simulink library "psa"  (R2021b)
settings: Solver=VariableStepAuto  StartTime=0.0  StopTime=10.0  RelTol=1e-3
undefined symbols (not defined in the file or in its folder): ENUM_B2VDCCHGCONNSTA_CONNECT, ENUM_BRAKEPEDAL_PRESSED, ENUM_HVPWROFFREQ_POWEROFF, ENUM_KEYSTATUS_OFF, ENUM_KEYSTATUS_ON, ENUM_KEYSTATUS_START, ENUM_MCUFAILGRADE_SEVERE, ENUM_PEUHVILSTA_EACERROR, ENUM_PEUHVILSTA_EHPSERROR, ENUM_PEUHVILSTA_PEUERROR, ENUM_PEUSELFCHKSTS_FAULT, ENUM_PMMMODE_INITIALIZE, ENUM_TARGETGEAR_NEUTRAL, FALSE, KPMM_ChrgwakeDebon_cnt, KPSA_ActTimeEmergencySD_s, KPSA_AfterrunWaitTime_s, KPSA_AlcLockPass_ovrdflg_flg, KPSA_AlcLockPass_ovrdval_flg, KPSA_AlcLockPassTime_s, KPSA_APSPosnSafe_pct, KPSA_FakeWakeRESET_flg, KPSA_Keystatus_enum_dovrdflg, KPSA_Keystatus_enum_dovrdval, KPSA_KeystatusWaitTime_s, KPSA_PBOnTimeForEMStop_s, KPSA_PBTrigHoldtime_s, KPSA_RcvTimeEmergencySD_s, KPSA_VehspdSafe_kph, TRUE
libraries: hcu_lib x7, simulink x3
settings Model: Creator=Shawn  LastModifiedBy=FVT22063
settings SolverCC: AlgebraicLoopSolver=TrustRegion
settings DebuggingCC: SFMachineParentedDataDiag=warning

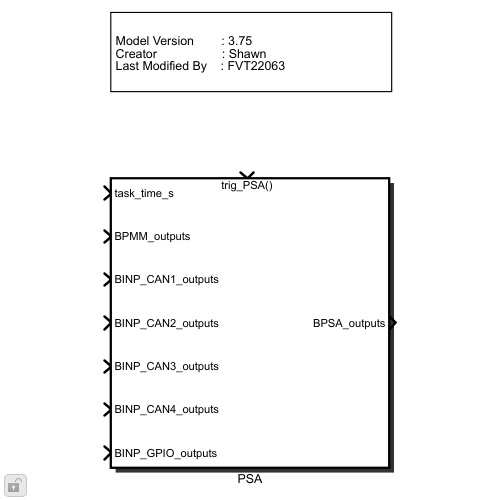
[thumbnail: Simulink's stored preview of the top-level diagram]
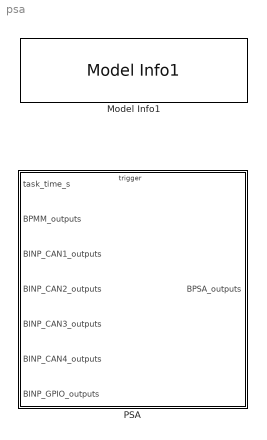
== system psa ==
  Model Info1 : hcu_lib/Model Info1  BlockCM=None  Frame=on  DisplayStringWithTags=|  HorizontalTextAlignment=Left  LeftAlignmentValue=0.02  SourceBlockDiagram=hcu_lib  TagMaxNumber=20
      | Model Version        : %<ModelVersion>
      | Creator                   : %<Creator>
      | Last Modified By    : %<LastModifiedBy>
      settings: SourceProductName=HCU Relative Block Library
  PSA : Subsystem
      settings: RTWSystemCode=Nonreusable function  RTWFcnNameOpts=Use subsystem name  RTWFileNameOpts=Use subsystem name

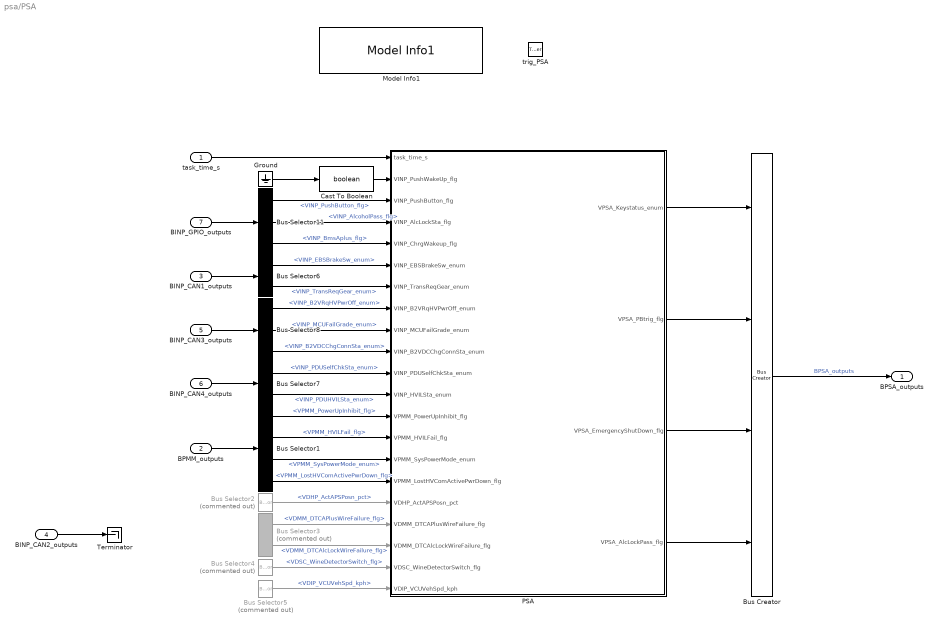
== system psa/PSA ==
  task_time_s : Inport
  BPMM_outputs : Inport  Port=2  OutDataTypeStr=Bus: BPMM_outputs
  BINP_CAN1_outputs : Inport  Port=3  OutDataTypeStr=Bus: BINP_CAN1_outputs
  BINP_CAN2_outputs : Inport  Port=4  OutDataTypeStr=Bus: BHAL_CAN2_outputs
  BINP_CAN3_outputs : Inport  Port=5  OutDataTypeStr=Bus: BINP_CAN3_outputs
  BINP_CAN4_outputs : Inport  Port=6  OutDataTypeStr=Bus: BINP_CAN4_outputs
  BINP_GPIO_outputs : Inport  Port=7  OutDataTypeStr=Bus: BINP_GPIO_outputs
  trig_PSA : TriggerPort  TriggerType=function-call  VariantControl=(inherit)
  Bus Creator : BusCreator  Inputs=4  OutDataTypeStr=Bus: BPSA_outputs  NonVirtualBus=on
  Bus Selector1 : BusSelector  OutputSignals=VPMM_PowerUpInhibit_flg,VPMM_HVILFail_flg,VPMM_SysPowerMode_enum,VPMM_LostHVComActivePwrDown_flg
  Bus Selector11 : BusSelector  OutputSignals=VINP_PushButton_flg,VINP_AlcoholPass_flg,VINP_BmsAplus_flg
  Bus Selector2 : BusSelector  Commented=on  OutputSignals=VDHP_ActAPSPosn_pct
  Bus Selector3 : BusSelector  Commented=on  OutputSignals=VDMM_DTCAPlusWireFailure_flg,VDMM_DTCAlcLockWireFailure_flg
  Bus Selector4 : BusSelector  Commented=on  OutputSignals=VDSC_WineDetectorSwitch_flg
  Bus Selector5 : BusSelector  Commented=on  OutputSignals=VDIP_VCUVehSpd_kph
  Bus Selector6 : BusSelector  OutputSignals=VINP_EBSBrakeSw_enum,VINP_TransReqGear_enum
  Bus Selector7 : BusSelector  OutputSignals=VINP_PDUSelfChkSta_enum,VINP_PDUHVILSta_enum
  Bus Selector8 : BusSelector  OutputSignals=VINP_B2VRqHVPwrOff_enum,VINP_MCUFailGrade_enum,VINP_B2VDCChgConnSta_enum
  Cast To Boolean : DataTypeConversion  OutDataTypeStr=boolean
  Ground : Ground
  Model Info1 : hcu_lib/Model Info1  BlockCM=None  Frame=on  DisplayStringWithTags=|  HorizontalTextAlignment=Left  LeftAlignmentValue=0.02  SourceBlockDiagram=hcu_lib  TagMaxNumber=20
      | Model Version        : %<ModelVersion>
      | Creator                   : %<Creator>
      | Last Modified By    : %<LastModifiedBy>
      settings: SourceProductName=HCU Relative Block Library
  PSA : Subsystem
  Terminator : Terminator
  BPSA_outputs : Outport  OutDataTypeStr=Bus: BPSA_outputs  VectorParamsAs1DForOutWhenUnconnected=off
  wires:
  Bus Selector1/1 -> PSA/13(VPMM_PowerUpInhibit_flg)  "<VPMM_PowerUpInhibit_flg>"
  Bus Creator/1 -> BPSA_outputs/1  "BPSA_outputs"
  PSA/1(VPSA_Keystatus_enum) -> Bus Creator/1
  task_time_s/1 -> PSA/1(task_time_s)
  PSA/2(VPSA_PBtrig_flg) -> Bus Creator/2
  PSA/3(VPSA_EmergencyShutDown_flg) -> Bus Creator/3
  Bus Selector2/1 -> PSA/17(VDHP_ActAPSPosn_pct)  "<VDHP_ActAPSPosn_pct>"
  Bus Selector1/2 -> PSA/14(VPMM_HVILFail_flg)  "<VPMM_HVILFail_flg>"
  PSA/4(VPSA_AlcLockPass_flg) -> Bus Creator/4
  Bus Selector1/3 -> PSA/15(VPMM_SysPowerMode_enum)  "<VPMM_SysPowerMode_enum>"
  Bus Selector1/4 -> PSA/16(VPMM_LostHVComActivePwrDown_flg)  "<VPMM_LostHVComActivePwrDown_flg>"
  Bus Selector3/1 -> PSA/18(VDMM_DTCAPlusWireFailure_flg)  "<VDMM_DTCAPlusWireFailure_flg>"
  Bus Selector3/2 -> PSA/19(VDMM_DTCAlcLockWireFailure_flg)  "<VDMM_DTCAlcLockWireFailure_flg>"
  Bus Selector4/1 -> PSA/20(VDSC_WineDetectorSwitch_flg)  "<VDSC_WineDetectorSwitch_flg>"
  Bus Selector5/1 -> PSA/21(VDIP_VCUVehSpd_kph)  "<VDIP_VCUVehSpd_kph>"
  BPMM_outputs/1 -> Bus Selector1/1
  BINP_CAN1_outputs/1 -> Bus Selector6/1
  Bus Selector6/1 -> PSA/6(VINP_EBSBrakeSw_enum)  "<VINP_EBSBrakeSw_enum>"
  BINP_CAN4_outputs/1 -> Bus Selector7/1
  Bus Selector7/2 -> PSA/12(VINP_HVILSta_enum)  "<VINP_PDUHVILSta_enum>"
  BINP_CAN3_outputs/1 -> Bus Selector8/1
  Bus Selector7/1 -> PSA/11(VINP_PDUSelfChkSta_enum)  "<VINP_PDUSelfChkSta_enum>"
  Bus Selector8/1 -> PSA/8(VINP_B2VRqHVPwrOff_enum)  "<VINP_B2VRqHVPwrOff_enum>"
  Bus Selector8/2 -> PSA/9(VINP_MCUFailGrade_enum)  "<VINP_MCUFailGrade_enum>"
  Bus Selector8/3 -> PSA/10(VINP_B2VDCChgConnSta_enum)  "<VINP_B2VDCChgConnSta_enum>"
  Bus Selector6/2 -> PSA/7(VINP_TransReqGear_enum)  "<VINP_TransReqGear_enum>"
  Ground/1 -> Cast To Boolean/1
  Cast To Boolean/1 -> PSA/2(VINP_PushWakeUp_flg)
  BINP_GPIO_outputs/1 -> Bus Selector11/1
  Bus Selector11/1 -> PSA/3(VINP_PushButton_flg)  "<VINP_PushButton_flg>"
  Bus Selector11/2 -> PSA/4(VINP_AlcLockSta_flg)  "<VINP_AlcoholPass_flg>"
  BINP_CAN2_outputs/1 -> Terminator/1
  Bus Selector11/3 -> PSA/5(VINP_ChrgWakeup_flg)  "<VINP_BmsAplus_flg>"

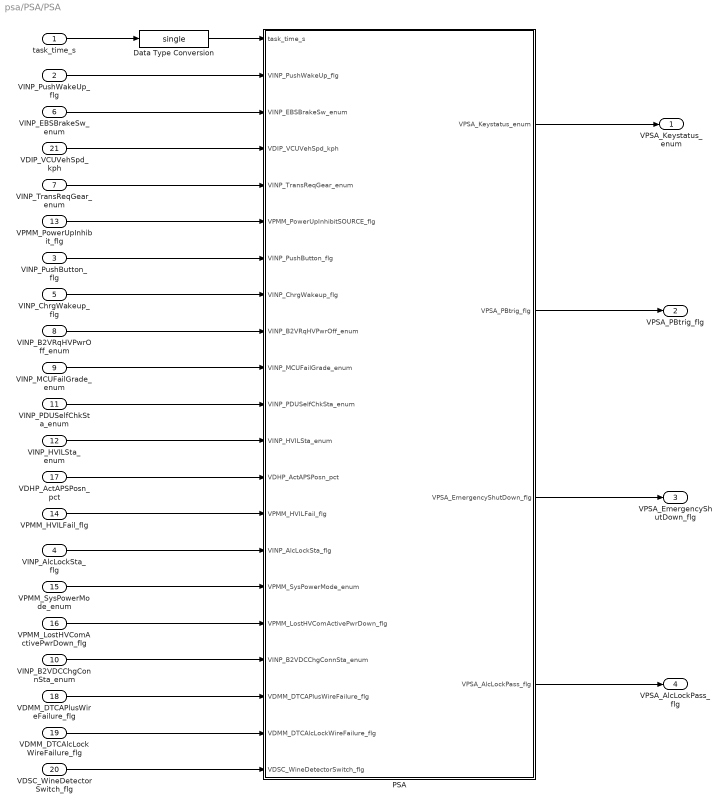
== system psa/PSA/PSA ==
  task_time_s : Inport
  VINP_PushWakeUp_flg : Inport  Port=2
  VINP_PushButton_flg : Inport  Port=3
  VINP_AlcLockSta_flg : Inport  Port=4
  VINP_ChrgWakeup_flg : Inport  Port=5
  VINP_EBSBrakeSw_enum : Inport  Port=6
  VINP_TransReqGear_enum : Inport  Port=7
  VINP_B2VRqHVPwrOff_enum : Inport  Port=8
  VINP_MCUFailGrade_enum : Inport  Port=9
  VINP_B2VDCChgConnSta_enum : Inport  Port=10
  VINP_PDUSelfChkSta_enum : Inport  Port=11
  VINP_HVILSta_enum : Inport  Port=12
  VPMM_PowerUpInhibit_flg : Inport  Port=13
  VPMM_HVILFail_flg : Inport  Port=14
  VPMM_SysPowerMode_enum : Inport  Port=15
  VPMM_LostHVComActivePwrDown_flg : Inport  Port=16
  VDHP_ActAPSPosn_pct : Inport  Port=17
  VDMM_DTCAPlusWireFailure_flg : Inport  Port=18
  VDMM_DTCAlcLockWireFailure_flg : Inport  Port=19
  VDSC_WineDetectorSwitch_flg : Inport  Port=20
  VDIP_VCUVehSpd_kph : Inport  Port=21
  Data Type Conversion : DataTypeConversion  OutDataTypeStr=single
  PSA : Subsystem  Priority=1
      settings: AttributesFormatString=< Priority = %<Priority>>
  VPSA_Keystatus_enum : Outport  VectorParamsAs1DForOutWhenUnconnected=off
  VPSA_PBtrig_flg : Outport  Port=2  VectorParamsAs1DForOutWhenUnconnected=off
  VPSA_EmergencyShutDown_flg : Outport  Port=3  VectorParamsAs1DForOutWhenUnconnected=off
  VPSA_AlcLockPass_flg : Outport  Port=4  VectorParamsAs1DForOutWhenUnconnected=off
  wires:
  VPMM_PowerUpInhibit_flg/1 -> PSA/6(VPMM_PowerUpInhibitSOURCE_flg)
  PSA/1(VPSA_Keystatus_enum) -> VPSA_Keystatus_enum/1
  VINP_PushWakeUp_flg/1 -> PSA/2(VINP_PushWakeUp_flg)
  VINP_TransReqGear_enum/1 -> PSA/5(VINP_TransReqGear_enum)
  VDIP_VCUVehSpd_kph/1 -> PSA/4("VDIP_VCUVehSpd_kph ")
  Data Type Conversion/1 -> PSA/1(task_time_s)
  VINP_PushButton_flg/1 -> PSA/7(VINP_PushButton_flg)
  VINP_EBSBrakeSw_enum/1 -> PSA/3(VINP_EBSBrakeSw_enum)
  task_time_s/1 -> Data Type Conversion/1
  VINP_ChrgWakeup_flg/1 -> PSA/8(VINP_ChrgWakeup_flg)
  PSA/2(VPSA_PBtrig_flg) -> VPSA_PBtrig_flg/1
  PSA/3(VPSA_EmergencyShutDown_flg) -> VPSA_EmergencyShutDown_flg/1
  VINP_B2VRqHVPwrOff_enum/1 -> PSA/9(VINP_B2VRqHVPwrOff_enum)
  VINP_PDUSelfChkSta_enum/1 -> PSA/11(VINP_PDUSelfChkSta_enum)
  VINP_HVILSta_enum/1 -> PSA/12(VINP_HVILSta_enum)
  VDHP_ActAPSPosn_pct/1 -> PSA/13(VDHP_ActAPSPosn_pct)
  VPMM_HVILFail_flg/1 -> PSA/14(VPMM_HVILFail_flg)
  VINP_MCUFailGrade_enum/1 -> PSA/10(VINP_MCUFailGrade_enum)
  VINP_AlcLockSta_flg/1 -> PSA/15(VINP_AlcLockSta_flg)
  PSA/4(VPSA_AlcLockPass_flg) -> VPSA_AlcLockPass_flg/1
  VPMM_SysPowerMode_enum/1 -> PSA/16(VPMM_SysPowerMode_enum)
  VPMM_LostHVComActivePwrDown_flg/1 -> PSA/17(VPMM_LostHVComActivePwrDown_flg)
  VINP_B2VDCChgConnSta_enum/1 -> PSA/18(VINP_B2VDCChgConnSta_enum)
  VDMM_DTCAPlusWireFailure_flg/1 -> PSA/19(VDMM_DTCAPlusWireFailure_flg)
  VDMM_DTCAlcLockWireFailure_flg/1 -> PSA/20(VDMM_DTCAlcLockWireFailure_flg)
  VDSC_WineDetectorSwitch_flg/1 -> PSA/21(VDSC_WineDetectorSwitch_flg)

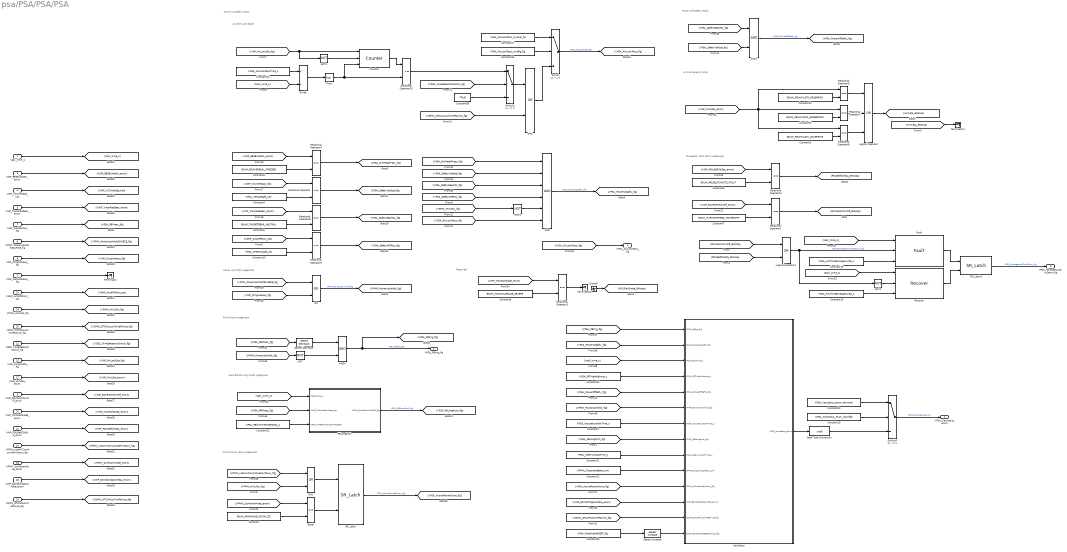
== system psa/PSA/PSA/PSA ==
  note: Push Button Judgement
  note: Active Power Down Judgement
  note: Emergency Shut Down Judgement
  note: Power Off Safety Check
  note: Reserved
  note: Push Botton Long Press Judgement
  note: Power Up Inhibit Judgement
  note: HVIL Emergency Stop
  note: Alcohol Lock State
  note: Power Up Safety Check
  task_time_s : Inport
  VINP_PushWakeUp_flg : Inport  Port=2
  VINP_EBSBrakeSw_enum : Inport  Port=3
  "VDIP_VCUVehSpd_kph " : Inport  Port=4
  VINP_TransReqGear_enum : Inport  Port=5
  VPMM_PowerUpInhibitSOURCE_flg : Inport  Port=6
  VINP_PushButton_flg : Inport  Port=7
  VINP_ChrgWakeup_flg : Inport  Port=8
  VINP_B2VRqHVPwrOff_enum : Inport  Port=9
  VINP_MCUFailGrade_enum : Inport  Port=10
  VINP_PDUSelfChkSta_enum : Inport  Port=11
  VINP_HVILSta_enum : Inport  Port=12
  VDHP_ActAPSPosn_pct : Inport  Port=13
  VPMM_HVILFail_flg : Inport  Port=14
  VINP_AlcLockSta_flg : Inport  Port=15
  VPMM_SysPowerMode_enum : Inport  Port=16
  VPMM_LostHVComActivePwrDown_flg : Inport  Port=17
  VINP_B2VDCChgConnSta_enum : Inport  Port=18
  VDMM_DTCAPlusWireFailure_flg : Inport  Port=19
  VDMM_DTCAlcLockWireFailure_flg : Inport  Port=20
  VDSC_WineDetectorSwitch_flg : Inport  Port=21
  AND : Logic  Inputs=6  AllPortsSameDT=off  OutDataTypeStr=boolean
  AND4 : Logic  AllPortsSameDT=off  OutDataTypeStr=boolean
  AND7 : Logic  AllPortsSameDT=off  OutDataTypeStr=boolean
  Constant : Constant  Value=ENUM_PMMMODE_INITIALIZE
  Constant1 : Constant  Value=KPSA_KeystatusWaitTime_s
  Constant10 : Constant  Value=ENUM_PEUHVILSTA_PEUERROR
  Constant11 : Constant  Value=KPSA_AfterrunWaitTime_s
  Constant12 : Constant  Value=KPMM_ChrgwakeDebon_cnt
  Constant13 : Constant  Value=KPSA_APSPosnSafe_pct
  Constant14 : Constant  Value=KPSA_AlcLockPassTime_s
  Constant15 : Constant  Value=KPSA_ActTimeEmergencySD_s
  Constant16 : Constant  Value=KPSA_AlcLockPass_ovrdflg_flg
  Constant17 : Constant  Value=KPSA_AlcLockPass_ovrdval_flg
  Constant18 : Constant  Value=KPSA_RcvTimeEmergencySD_s
  Constant19 : Constant  Value=KPSA_Keystatus_enum_dovrdflg
  Constant2 : Constant  Value=ENUM_PEUHVILSTA_EHPSERROR
  Constant20 : Constant  Value=KPSA_Keystatus_enum_dovrdval
  Constant21 : Constant  Value=KPSA_PBTrigHoldtime_s
  Constant22 : Constant  Value=KPSA_PBOnTimeForEMStop_s
  Constant23 : Constant  Value=KPSA_FakeWakeRESET_flg
  Constant3 : Constant  Value=ENUM_PEUHVILSTA_EACERROR
  Constant4 : Constant  Value=KPSA_VehspdSafe_kph
  Constant5 : Constant  Value=ENUM_TARGETGEAR_NEUTRAL
  Constant58 : Constant  Value=TRUE
  Constant6 : Constant  Value=ENUM_BRAKEPEDAL_PRESSED
  Constant7 : Constant  Value=ENUM_HVPWROFFREQ_POWEROFF
  Constant8 : Constant  Value=ENUM_MCUFAILGRADE_SEVERE
  Constant9 : Constant  Value=ENUM_PEUSELFCHKSTS_FAULT
  Counter : hcu_lib/Basic_Blocks/Counter
      settings: SourceProductName=HCU Relative Block Library
  Data Type Conversion : DataTypeConversion  OutDataTypeStr=uint8
  Detect Decrease : simulink/Logic and Bit Operations/Detect Decrease  vinit=0.0  OutDataTypeStr=boolean
  Detect Increase : simulink/Logic and Bit Operations/Detect Increase  vinit=0.0  OutDataTypeStr=boolean
  Divide : Product  Inputs=*/
  Equal : RelationalOperator  Operator===  OutDataTypeStr=boolean  RndMeth=Simplest
  Fault : hcu_lib/Basic_Blocks/Fault  SystemSampleTime=-1  VariantActivationTime=update diagram  Latency=0  AutoFrameSizeCalculation=off
      settings: SourceProductName=HCU Relative Block Library
  Floor : Rounding
  Ground : Ground
  KeyStatus : Stateflow chart  TreatAsAtomicUnit=on
  Logical Operator : Logic  Operator=OR  Inputs=3  AllPortsSameDT=off  OutDataTypeStr=boolean
  Logical Operator1 : Logic  Operator=OR  AllPortsSameDT=off  OutDataTypeStr=boolean
  NOT{,1..3} (4 alike) : Logic  Operator=NOT  AllPortsSameDT=off  OutDataTypeStr=boolean
  OR : Logic  Operator=OR  AllPortsSameDT=off  OutDataTypeStr=boolean
  OR1 : Logic  Operator=OR  AllPortsSameDT=off  OutDataTypeStr=boolean
  OR2 : Logic  Operator=OR  AllPortsSameDT=off  OutDataTypeStr=boolean
  PBLongPush : Subsystem
  Recover : hcu_lib/Basic_Blocks/Recover  SystemSampleTime=-1  VariantActivationTime=update diagram  Latency=0  AutoFrameSizeCalculation=off
      settings: SourceProductName=HCU Relative Block Library
  Relational Operator : RelationalOperator  Operator=<=  OutDataTypeStr=boolean  RndMeth=Simplest
  Relational Operator{1..8} (8 alike) : RelationalOperator  Operator===  OutDataTypeStr=boolean  RndMeth=Simplest
  Relational Operator10 : RelationalOperator  OutDataTypeStr=boolean  RndMeth=Simplest
  Relational Operator9 : RelationalOperator  Operator=<=  OutDataTypeStr=boolean  RndMeth=Simplest
  SR_Latch : hcu_lib/Basic_Blocks/SR_Latch
      settings: SourceProductName=HCU Relative Block Library
  SR_Latch1 : hcu_lib/Basic_Blocks/SR_Latch
      settings: SourceProductName=HCU Relative Block Library
  Switch : Switch  Criteria=u2 ~= 0
      settings: AttributesFormatString=%<Criteria>
  Switch3 : Switch  Criteria=u2 ~= 0
      settings: AttributesFormatString=%<Criteria>
  Switch4 : Switch  Criteria=u2 ~= 0
      settings: AttributesFormatString=%<Criteria>
  Terminator : Terminator
  Terminator1 : Terminator
  Terminator2 : Terminator
  VPSA_Keystatus_enum : Outport
  VPSA_PBtrig_flg : Outport  Port=2
  VPSA_EmergencyShutDown_flg : Outport  Port=3
  VPSA_AlcLockPass_flg : Outport  Port=4
  wires:
  Relational Operator2/1 -> Terminator2/1
  KeyStatus/1(VPSA_Keystatus_enum) -> Data Type Conversion/1
  NOT/1 -> AND4/2
  [VPMM_PowerUpInhibit_flg] -> KeyStatus/6(VPMM_PowerUpInhibit_flg)
  PBLongPush/1(VPSA_PowerDownForEM_flg) -> [VPSA_PBLongPush_flg]  "VPSA_PBLongPush_flg"
  [VPSA_PBPress_flg] -> PBLongPush/2(VINP_PushbuttonPress_flg)
  Constant22/1 -> PBLongPush/3(KPSA_TIMEPushbuttonPressEM)
  [task_time_s] -> PBLongPush/1(Task_time_s)
  [VPSA_PowerOffSafty_flg] -> KeyStatus/5(VPSA_PowerOffSafty_flg)
  AND7/1 -> [VPSA_PowerOffSafty_flg]  "VPSA_PowerOffSafty_flg"
  [VPSA_SafetyVehSpd_flg] -> AND7/2
  [VPSA_SafetyGearPos_flg] -> AND7/1
  Constant21/1 -> KeyStatus/4(KPSA_PBTrigHoldtime_s)
  [task_time_s] -> KeyStatus/3(VPSA_tasktime_s)
  [VPSA_PowerUpSafty_flg] -> KeyStatus/2(VPSA_PowerUpSafty_flg)
  [VPSA_PBtrig_flg] -> KeyStatus/1(VPSA_PBtrig_flg)
  AND4/1 -> VPSA_PBtrig_flg/1, [VPSA_PBtrig_flg]  "VPSA_PBtrig_flg"
  [VPSA_PBPress_flg] -> Detect Decrease/1
  Detect Decrease/1 -> AND4/1
  [VPMM_PowerUpInhibit_flg] -> NOT/1
  AND/1 -> [VPSA_PowerUpSafty_flg]  "VPSA_PowerUpSafty_flg"
  [VPSA_SafetyGearPos_flg] -> AND/3
  [VPSA_SafetyVehSpd_flg] -> AND/2
  [VPSA_BrkPedalPress_flg] -> AND/1
  VINP_PushButton_flg/1 -> [VPSA_PBPress_flg]
  VINP_PushWakeUp_flg/1 -> Terminator/1
  Constant4/1 -> Relational Operator/2
  Constant6/1 -> Relational Operator4/2
  Constant5/1 -> Relational Operator6/2
  Relational Operator6/1 -> [VPSA_SafetyGearPos_flg]
  Relational Operator/1 -> [VPSA_SafetyVehSpd_flg]
  task_time_s/1 -> [task_time_s]
  Relational Operator4/1 -> [VPSA_BrkPedalPress_flg]
  Constant1/1 -> KeyStatus/7(KPSA_KeystatusWaitTime_s)
  Constant7/1 -> Relational Operator1/2
  Constant8/1 -> Relational Operator2/2
  Constant9/1 -> Relational Operator3/2
  Constant10/1 -> Relational Operator5/2
  Constant2/1 -> Relational Operator7/2
  Constant3/1 -> Relational Operator8/2
  Relational Operator1/1 -> [B2VRqHVPwrOff_EMstop]
  Relational Operator3/1 -> [PDUSelfChkSta_EMstop]
  Relational Operator7/1 -> Logical Operator/2
  Relational Operator5/1 -> Logical Operator/1
  Relational Operator8/1 -> Logical Operator/3
  Logical Operator/1 -> [HVILSta_EMstop]
  Logical Operator1/1 -> NOT2/1, Fault/2  "VPSA_EmergencyShutDown_flg"
  [VPSA_PBLongPush_flg] -> KeyStatus/8(VPSA_PBLongPush_flg)
  OR/1 -> [VPMM_PowerUpInhibit_flg]  "VPMM_PowerUpInhibit_flg"
  [PDUSelfChkSta_EMstop] -> Logical Operator1/2
  [B2VRqHVPwrOff_EMstop] -> Logical Operator1/1
  Constant11/1 -> KeyStatus/9(KPSA_AfterrunWaitTime_s)
  Constant12/1 -> KeyStatus/10(KPMM_ChrgwakeDebon_cnt)
  [HVILSta_EMstop] -> Terminator1/1
  VDHP_ActAPSPosn_pct/1 -> [VDHP_ActAPSPosn_pct]
  [VDHP_ActAPSPosn_pct] -> Relational Operator9/1
  Constant13/1 -> Relational Operator9/2
  Relational Operator9/1 -> [VPSA_SafetyAPSPos_flg]
  [VPSA_SafetyAPSPos_flg] -> AND/4
  VPMM_HVILFail_flg/1 -> [VPMM_HVILFail_flg]
  [VPMM_HVILFail_flg] -> OR1/2
  VINP_AlcLockSta_flg/1 -> [VINP_AlcLockSta_flg]
  [VINP_AlcLockSta_flg] -> NOT1/1, Counter/1
  NOT1/1 -> Counter/2
  Constant14/1 -> Divide/1
  [task_time_s] -> Divide/2
  Divide/1 -> Floor/1
  Floor/1 -> Counter/3, Relational Operator10/2
  Switch/1 -> [VPSA_AlcLockPass_flg]  "VPSA_AlcLockPass_flg"
  Constant16/1 -> Switch/2
  Constant17/1 -> Switch/1
  Counter/1 -> Relational Operator10/1
  Relational Operator10/1 -> Switch3/1
  Constant/1 -> Equal/2
  Equal/1 -> SR_Latch/2
  OR1/1 -> SR_Latch/1
  [task_time_s] -> Fault/1
  NOT2/1 -> Recover/2
  Fault/1 -> SR_Latch1/1
  Recover/1 -> SR_Latch1/2
  SR_Latch1/1 -> VPSA_EmergencyShutDown_flg/1  "VPSA_EmergencyShutDown_flg"
  Constant15/1 -> Fault/3
  Constant18/1 -> Recover/3
  [VPMM_HVILFail_flg] -> NOT3/1
  Switch4/1 -> VPSA_Keystatus_enum/1  "VPSA_Keystatus_enum"
  Data Type Conversion/1 -> Switch4/3
  Constant19/1 -> Switch4/2
  Constant20/1 -> Switch4/1
  VDMM_DTCAlcLockWireFailure_flg/1 -> [VDMM_DTCAlcLockWireFailure_flg]
  VDSC_WineDetectorSwitch_flg/1 -> [VDSC_WineDetectorSwitch_flg]
  NOT3/1 -> AND/5
  Constant58/1 -> Switch3/3
  Switch3/1 -> OR2/1
  [task_time_s] -> Recover/1
  VINP_EBSBrakeSw_enum/1 -> [VINP_EBSBrakeSw_enum]
  [VINP_EBSBrakeSw_enum] -> Relational Operator4/1
  "VDIP_VCUVehSpd_kph "/1 -> [VDIP_VCUVehSpd_kph]
  [VDIP_VCUVehSpd_kph] -> Relational Operator/1
  VINP_TransReqGear_enum/1 -> [VINP_TransReqGear_enum]
  [VINP_TransReqGear_enum] -> Relational Operator6/1
  [VPMM_PowerUpInhibitSOUECE_flg] -> OR/1
  VPMM_PowerUpInhibitSOURCE_flg/1 -> [VPMM_PowerUpInhibitSOUECE_flg]
  VINP_ChrgWakeup_flg/1 -> [VINP_ChrgWakeup_flg]
  [VINP_ChrgWakeup_flg] -> OR/2
  VINP_HVILSta_enum/1 -> [VINP_HVILSta_enum]
  [VINP_HVILSta_enum] -> Relational Operator8/1, Relational Operator7/1, Relational Operator5/1
  VINP_B2VRqHVPwrOff_enum/1 -> [VINP_B2VRqHVPwrOff_enum]
  [VINP_B2VRqHVPwrOff_enum] -> Relational Operator1/1
  VINP_MCUFailGrade_enum/1 -> [VINP_MCUFailGrade_enum]
  [VINP_MCUFailGrade_enum] -> Relational Operator2/1
  [VINP_PDUSelfChkSta_enum] -> Relational Operator3/1
  VINP_PDUSelfChkSta_enum/1 -> [VINP_PDUSelfChkSta_enum]
  [VPSA_AlcLockPass_flg] -> VPSA_AlcLockPass_flg/1
  Ground/1 -> [MCUFailGrade_EMstop]
  SR_Latch/1 -> [VPSA_ActivePowerDwon_flg]  "VPSA_ActivePowerDwon_flg"
  [VPSA_ActivePowerDwon_flg] -> KeyStatus/11(VPSA_ActivePowerDwon_flg)
  VPMM_LostHVComActivePwrDown_flg/1 -> [VPMM_LostHVComActivePwrDown_flg]
  [VPMM_LostHVComActivePwrDown_flg] -> OR1/1
  VPMM_SysPowerMode_enum/1 -> [VPMM_SysPowerMode_enum]
  [VPMM_SysPowerMode_enum] -> Equal/1
  VINP_B2VDCChgConnSta_enum/1 -> [VINP_B2VDCChgConnSta_enum]
  [VINP_B2VDCChgConnSta_enum] -> KeyStatus/12(VINP_B2VDCChgConnSta_enum)
  VDMM_DTCAPlusWireFailure_flg/1 -> [VDMM_DTCAPlusWireFailure_flg]
  [VDMM_DTCAPlusWireFailure_flg] -> KeyStatus/13(VDMM_DTCAPlusWireFailure_flg)
  [VDMM_DTCAlcLockWireFailure_flg] -> OR2/2
  [VDSC_WineDetectorSwitch_flg] -> Switch3/2
  OR2/1 -> Switch/3
  [VPSA_AlcLockPass_flg] -> AND/6
  Constant23/1 -> Detect Increase/1
  Detect Increase/1 -> KeyStatus/14(KPSA_FakeWakeRESETRising_flg)

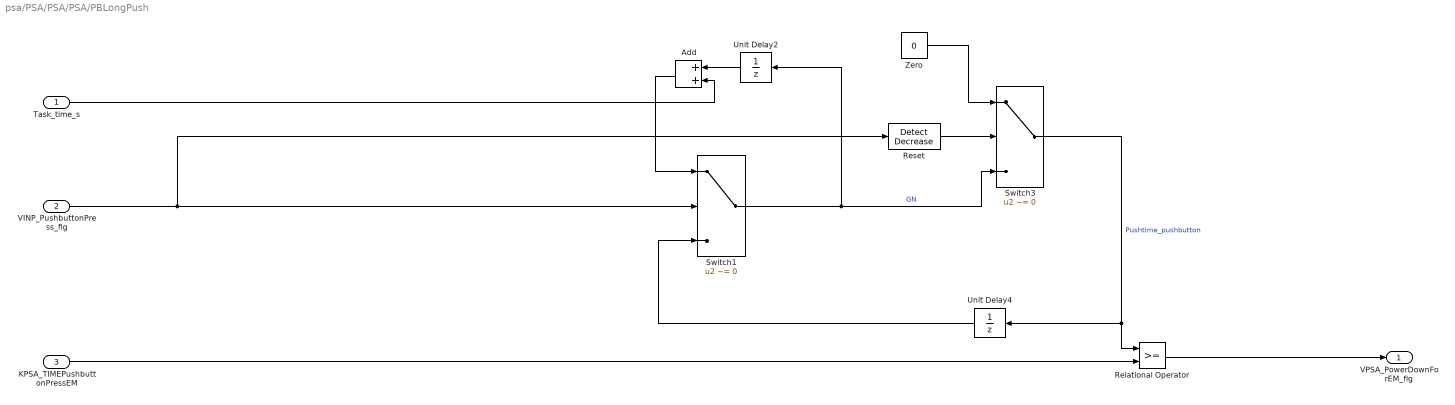
== system psa/PSA/PSA/PSA/PBLongPush ==
  Task_time_s : Inport
  VINP_PushbuttonPress_flg : Inport  Port=2
  KPSA_TIMEPushbuttonPressEM : Inport  Port=3
  Add : Sum
  Relational Operator : RelationalOperator  OutDataTypeStr=boolean  RndMeth=Simplest
  Reset : simulink/Logic and Bit Operations/Detect Decrease  vinit=0.0  OutDataTypeStr=boolean
  Switch1 : Switch  Criteria=u2 ~= 0  Threshold=2
  Switch3 : Switch  Criteria=u2 ~= 0  Threshold=2
  Unit Delay2 : UnitDelay  SampleTime=-1  HasFrameUpgradeWarning=on
  Unit Delay4 : UnitDelay  SampleTime=-1  HasFrameUpgradeWarning=on
  Zero : Constant  Value=0
  VPSA_PowerDownForEM_flg : Outport  VectorParamsAs1DForOutWhenUnconnected=off
  wires:
  Switch1/1 -> Unit Delay2/1, Switch3/3  "GN"
  Task_time_s/1 -> Add/2
  Relational Operator/1 -> VPSA_PowerDownForEM_flg/1
  Switch3/1 -> Relational Operator/1, Unit Delay4/1  "Pushtime_pushbutton"
  Unit Delay4/1 -> Switch1/3
  Reset/1 -> Switch3/2
  VINP_PushbuttonPress_flg/1 -> Switch1/2, Reset/1
  Add/1 -> Switch1/1
  Unit Delay2/1 -> Add/1
  Zero/1 -> Switch3/1
  KPSA_TIMEPushbuttonPressEM/1 -> Relational Operator/2

== stateflow chart psa/PSA/PSA/PSA/KeyStatus ==
  state Boot
    en:
    VPSA_Keystatus_enum = ENUM_KEYSTATUS_OFF;
    du:
    VPMM_ChrgwakeDebon_cnt += 1;
  state Execution
    state _1stPress
      en:
      VPSA_KeyStateChk_flg = FALSE;
      (default) -> (junction 27) : {
          | VPSA_TimeWaitForChk_s = 0;
          | }
      _1stPress -> (junction 27) [order 1]
      (junction 27) -> (junction 31) [order 1] : [(VPSA_PowerUpSafty_flg)&&(VPSA_TimeWaitForChk_s < KPSA_PBTrigHoldtime_s) ]
      (junction 27) -> (junction 61) [order 2] : {
          | VPSA_TimeWaitForChk_s = VPSA_TimeWaitForChk_s+ VPSA_tasktime_s;
          | VPSA_Keystatus_enum = ENUM_KEYSTATUS_ON;
          | }
      (junction 31) -> (junction 60) : {
          | VPSA_KeyStateChk_flg = TRUE;
          | VPSA_TimeWaitForChk_s = 0;
          | }
      (junction 60) -> (junction 61)
    state ON
      en:
      VPSA_Keystatus_enum = ENUM_KEYSTATUS_ON;
      VPSA_TimeWaitForChk_s = 0 ;
      (default) -> (junction 77) : {VPSA_ONWaitTimer_s = 0;
          |  VPSA_ONTimeout_flg = FALSE;}
      ON -> (junction 77) [order 1]
      (junction 77) -> (junction 165) [order 1] : [VPSA_ONWaitTimer_s > KPSA_KeystatusWaitTime_s]
      (junction 77) -> (junction 81) [order 2] : {
          | VPSA_ONWaitTimer_s = VPSA_ONWaitTimer_s+ VPSA_tasktime_s;
          | }
      (junction 165) -> (junction 167) : {VPSA_ONTimeout_flg = TRUE;}
      (junction 167) -> (junction 81)
    state START
      en:
      VPSA_Keystatus_enum = ENUM_KEYSTATUS_START;
      (default) -> (junction 158) : {VPSA_STARTWaitTimer_s = 0;
          |  VPSA_STARTTimeout_flg = FALSE;}
      START -> (junction 158) [order 1]
      (junction 158) -> (junction 160) [order 1] : [VPSA_STARTWaitTimer_s > KPSA_KeystatusWaitTime_s]
      (junction 158) -> (junction 85) [order 2] : {
          | VPSA_STARTWaitTimer_s = VPSA_STARTWaitTimer_s+ VPSA_tasktime_s;
          | }
      (junction 160) -> (junction 162) : {VPSA_STARTTimeout_flg = TRUE;}
      (junction 162) -> (junction 85)
    state OFF
      en:
      VPSA_Keystatus_enum = ENUM_KEYSTATUS_OFF;
      (default) -> (junction 91) : {VPSA_OFFWaitTimer_s = 0;
          |  VPSA_OFFTimeout_flg = FALSE;}
      OFF -> (junction 91) [order 1]
      (junction 91) -> (junction 170) [order 1] : [VPSA_OFFWaitTimer_s > KPSA_AfterrunWaitTime_s]
      (junction 91) -> (junction 90) [order 2] : {
          | VPSA_OFFWaitTimer_s = VPSA_OFFWaitTimer_s+ VPSA_tasktime_s;
          | }
      (junction 170) -> (junction 172) : {VPSA_OFFTimeout_flg = TRUE;}
      (junction 172) -> (junction 90)
    (default) -> _1stPress
    _1stPress -> ON [order 2] : [VPSA_TimeWaitForChk_s > KPSA_PBTrigHoldtime_s]
    _1stPress -> START [order 1] : [VPSA_KeyStateChk_flg]
    ON -> START [order 1] : [VPSA_PBtrig_flg&&...
        | VPSA_PowerUpSafty_flg]
    ON -> OFF [order 2] : [VPSA_ONTimeout_flg && ...
        | (VPSA_PBtrig_flg|| VPSA_PBLongPush_flg ||...
        | (VPMM_PowerUpInhibit_flg && (VDMM_DTCAPlusWireFailure_flg ||...
        | (VINP_B2VDCChgConnSta_enum == ENUM_B2VDCCHGCONNSTA_CONNECT))))]
    START -> OFF [order 1] : [(VPSA_STARTTimeout_flg && VPSA_PBtrig_flg && VPSA_PowerOffSafty_flg) || ...
        |  (VPSA_PBLongPush_flg) || (VPSA_ActivePowerDwon_flg && VPSA_PBtrig_flg) ]
    OFF -> ON [order 1] : [VPSA_OFFTimeout_flg && VPSA_PBtrig_flg]
  (default) -> Boot
  Boot -> Execution : [
      | VPMM_PowerUpInhibit_flg == FALSE &&...
      | VPMM_ChrgwakeDebon_cnt > KPMM_ChrgwakeDebon_cnt
      | ]
  Execution -> Boot : [KPSA_FakeWakeRESETRising_flg]
  data: VPSA_PBtrig_flg input; VPSA_PowerUpSafty_flg input; VPSA_tasktime_s input; KPSA_PBTrigHoldtime_s input; VPSA_PowerOffSafty_flg input; VPSA_Keystatus_enum output; VPSA_TimeWaitForChk_s local single; ENUM_KEYSTATUS_OFF parameter; ENUM_KEYSTATUS_ON parameter; ENUM_KEYSTATUS_START parameter; VPMM_PowerUpInhibit_flg input; VPSA_KeyStateChk_flg local boolean; FALSE parameter; TRUE parameter; VPSA_TimeWaitForTrig_s local single; KPSA_KeystatusWaitTime_s input; VPSA_PBLongPush_flg input; KPSA_AfterrunWaitTime_s input; KPMM_ChrgwakeDebon_cnt input; VPMM_ChrgwakeDebon_cnt local double; VPSA_ActivePowerDwon_flg input; VINP_B2VDCChgConnSta_enum input; VDMM_DTCAPlusWireFailure_flg input; ENUM_B2VDCCHGCONNSTA_CONNECT parameter; VPSA_STARTTimeout_flg local boolean; VPSA_STARTWaitTimer_s local single; VPSA_ONWaitTimer_s local single; VPSA_ONTimeout_flg local boolean; VPSA_OFFWaitTimer_s local single; VPSA_OFFTimeout_flg local boolean; KPSA_FakeWakeRESETRising_flg input boolean size=1
